simulink model "controller_lonHdot_for_bode"  (R2017b)
settings: Solver=VariableStepAuto  StartTime=0.0  StopTime=30  RelTol=1e-3
values from neighbouring files (symbols this model uses):
  CSim_Hdot = 1    [controller_lonHdot_design.m]
  KF_Hdot = 0    [controller_lonHdot_design.m]
  KF_theta = 0    [controller_lonHdot_design.m]
  KI_Hdot = 0    [controller_lonHdot_design.m]
  KI_theta = 0    [controller_lonHdot_design.m]
  KP_Hdot = 1    [controller_lonHdot_design.m]
  KP_q = 1    [controller_lonHdot_design.m]
  KP_q2 = 1    [controller_lonHdot_design.m]
  KP_theta = 1    [controller_lonHdot_design.m]
  Tau_DE = 0.05    [controller_lonHdot_design.m]
undefined symbols (not defined in the file or in its folder): Actuators, Linmod
settings Model: Creator=zht  LastModifiedBy=zht

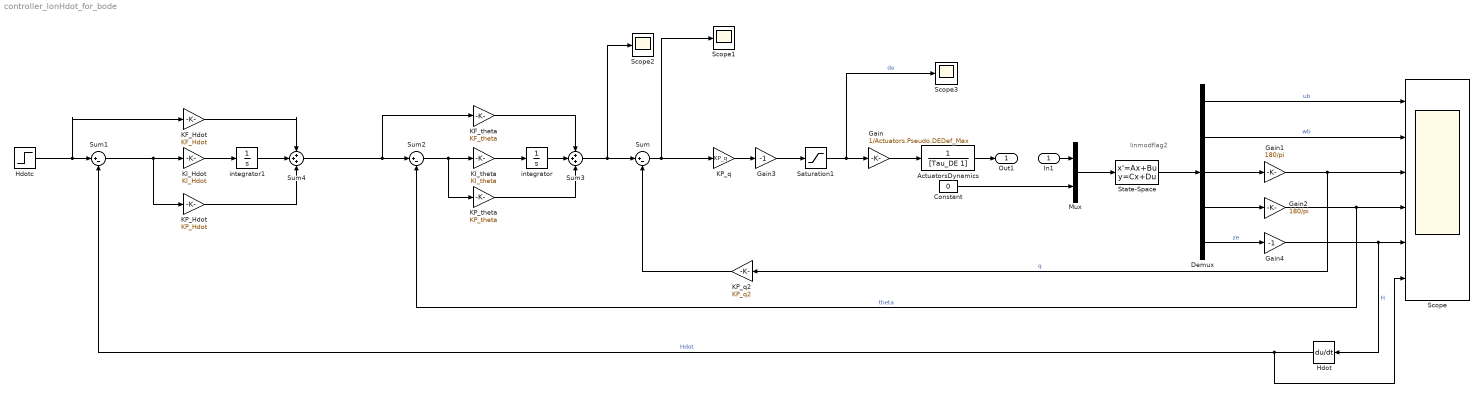
== system controller_lonHdot_for_bode ==
  note: linmodflag2
  In1 : Inport
  ActuatorsDynamics : TransferFcn  Denominator=[Tau_DE 1]
  Constant : Constant  Value=0
  Demux : Demux  Outputs=5
  Gain : Gain  Gain=1/Actuators.Pseudo.DEDef_Max
  Gain1 : Gain  Gain=180/pi
  Gain2 : Gain  Gain=180/pi
  Gain3 : Gain  Gain=-1
  Gain4 : Gain  Gain=-1
  Hdot : Derivative  CoefficientInTFapproximation=0.0001
  Hdotc : Step  Time=0  After=CSim_Hdot  SampleTime=0
  KF_Hdot : Gain  Gain=KF_Hdot
  KF_theta : Gain  Gain=KF_theta
  KI_Hdot : Gain  Gain=KI_Hdot
  KI_theta : Gain  Gain=KI_theta
  KP_Hdot : Gain  Gain=KP_Hdot
  KP_q : Gain  Gain=KP_q
  KP_q2 : Gain  Gain=KP_q2
  KP_theta : Gain  Gain=KP_theta
  Mux : Mux  Inputs=2
  Saturation1 : Saturate  UpperLimit=Actuators.Pseudo.DEDef_Max  LowerLimit=-Actuators.Pseudo.DEDef_Max
  Scope : Scope  NumInputPorts=6
  Scope1 : Scope
  Scope2 : Scope
  Scope3 : Scope
  State-Space : StateSpace  A=Linmod.Lon_5.A  B=Linmod.Lon_5.B  C=Linmod.Lon_5.C  D=Linmod.Lon_5.D  InitialCondition=0  ContinuousStateAttributes={'ub','wb','q','theta','H'}
  Sum : Sum  Inputs=|+-
  Sum1 : Sum  Inputs=|+-
  Sum2 : Sum  Inputs=|+-
  Sum3 : Sum  Inputs=+++
  Sum4 : Sum  Inputs=+++
  integrator : Integrator
  integrator1 : Integrator
  Out1 : Outport
  wires:
  Mux/1 -> State-Space/1
  Constant/1 -> Mux/2
  State-Space/1 -> Demux/1
  Demux/2 -> Scope/2  "wb"
  Demux/3 -> Gain1/1
  Demux/4 -> Gain2/1
  Demux/5 -> Gain4/1  "ze"
  Demux/1 -> Scope/1  "ub"
  Gain1/1 -> KP_q2/1, Scope/3  "q"
  Gain2/1 -> Sum2/2, Scope/4  "theta"
  Gain/1 -> ActuatorsDynamics/1
  Sum/1 -> KP_q/1, Scope1/1
  Sum3/1 -> Scope2/1, Sum/1
  Sum2/1 -> KP_theta/1, KI_theta/1
  KP_q2/1 -> Sum/2
  Saturation1/1 -> Scope3/1, Gain/1  "de"
  Gain3/1 -> Saturation1/1
  Sum1/1 -> KP_Hdot/1, KI_Hdot/1
  KP_q/1 -> Gain3/1
  integrator/1 -> Sum3/2
  KF_theta/1 -> Sum3/1
  KP_theta/1 -> Sum3/3
  KI_theta/1 -> integrator/1
  Hdot/1 -> Scope/6, Sum1/2  "Hdot"
  Sum4/1 -> KF_theta/1, Sum2/1
  KI_Hdot/1 -> integrator1/1
  Hdotc/1 -> KF_Hdot/1, Sum1/1
  KP_Hdot/1 -> Sum4/3
  integrator1/1 -> Sum4/2
  KF_Hdot/1 -> Sum4/1
  Gain4/1 -> Hdot/1, Scope/5  "H"
  ActuatorsDynamics/1 -> Out1/1
  In1/1 -> Mux/1
